simulink model "untitled"  (R2020b)
settings: Solver=ode1  StartTime=0  StopTime=max(T)  FixedStep=0.01  RelTol=1e-3
values from neighbouring files (symbols this model uses):
  H = [0 costh 0 ... (first row only)    [kalmanf_unbias.m]
  P0 = [10000 5000 5000 ... (first row only)    [Kalman.m]
  Q = [100 50 25 ... (first row only)    [Kalman.m]
  R = [10 5 5 ... (first row only)    [Kalman.m]
  x0 = zeros(3,1)    [Kalman.m]
settings Model: Creator=Stergios  LastModifiedBy=Stergios

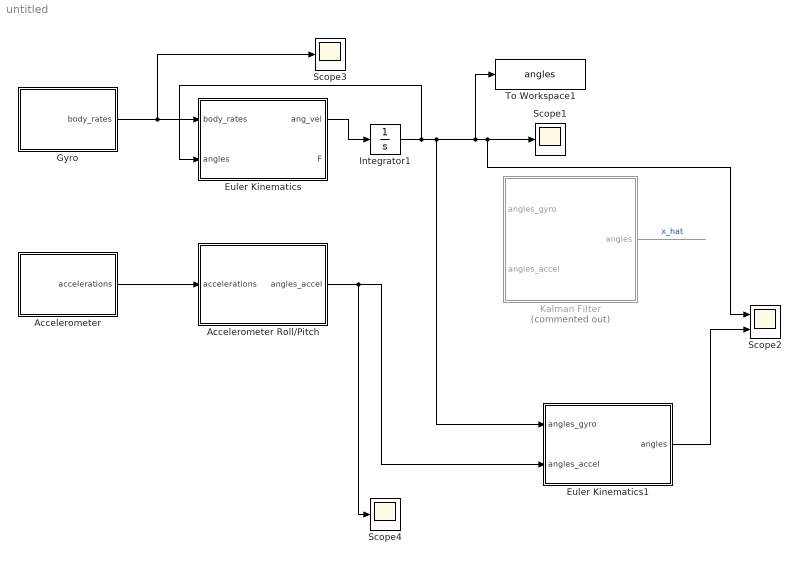
== system untitled ==
  Accelerometer : Subsystem
  Accelerometer Roll/Pitch : MATLAB Function  TreatAsAtomicUnit=on
  Euler Kinematics : MATLAB Function  TreatAsAtomicUnit=on
  Euler Kinematics1 : MATLAB Function  TreatAsAtomicUnit=on
  Gyro : Subsystem
  Integrator1 : Integrator  InitialCondition=[0 0 0]
  Kalman Filter : MATLAB Function  Commented=on  TreatAsAtomicUnit=on  mask{x0=x0, P0=P0, Q=Q, R=R, H=H}
      mask prompts: x0 "Initial State:"; P0 "Initial State Covariance Matrix:"; Q "Process Noise Covariance Matrix:"; R "Measurement Noise Covariance Matrix:"; H "Observation Matrix:"
  Scope1 : Scope
  Scope2 : Scope  NumInputPorts=2
  Scope3 : Scope
  Scope4 : Scope
  To Workspace1 : ToWorkspace  VariableName=angles  SampleTime=-1
  wires:
  Integrator1/1 -> Euler Kinematics1/1(angles_gyro), Scope1/1, Scope2/1, To Workspace1/1, Euler Kinematics/2(angles)
  Euler Kinematics/1(ang_vel) -> Integrator1/1
  Gyro/1(body_rates) -> Scope3/1, Euler Kinematics/1(body_rates)
  Accelerometer/1(accelerations) -> Accelerometer Roll/Pitch/1(accelerations)
  Kalman Filter/1(angles) -> ?  "x_hat"
  Euler Kinematics1/1(angles) -> Scope2/2
  Accelerometer Roll/Pitch/1(angles_accel) -> Scope4/1, Euler Kinematics1/2(angles_accel)

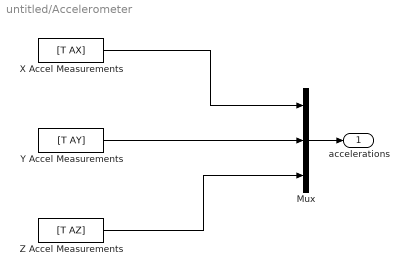
== system untitled/Accelerometer ==
  Mux : Mux  Inputs=3
  X Accel Measurements : FromWorkspace  VariableName=[T AX]
  Y Accel Measurements : FromWorkspace  VariableName=[T AY]
  Z Accel Measurements : FromWorkspace  VariableName=[T AZ]
  accelerations : Outport
  wires:
  Y Accel Measurements/1 -> Mux/2
  Z Accel Measurements/1 -> Mux/3
  Mux/1 -> accelerations/1
  X Accel Measurements/1 -> Mux/1

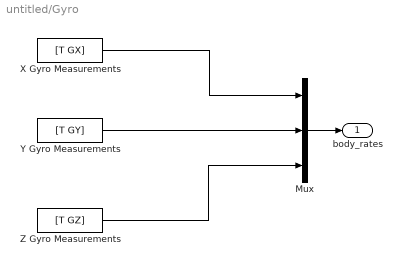
== system untitled/Gyro ==
  Mux : Mux  Inputs=3
  X Gyro Measurements : FromWorkspace  VariableName=[T GX]
  Y Gyro Measurements : FromWorkspace  VariableName=[T GY]
  Z Gyro Measurements : FromWorkspace  VariableName=[T GZ]
  body_rates : Outport
  wires:
  Mux/1 -> body_rates/1
  X Gyro Measurements/1 -> Mux/1
  Y Gyro Measurements/1 -> Mux/2
  Z Gyro Measurements/1 -> Mux/3

== matlab function untitled/Euler Kinematics ==
  data: body_rates input; ang_vel output; angles input; F output
function [ang_vel,F]=fcn(body_rates,angles)
    phi = angles(1)*pi/180;
    theta = angles(2)*pi/180;
    
    F = [1,tan(theta)*sin(phi),tan(theta)*cos(phi);
        0,cos(phi),-sin(phi);
        0,sin(phi)/cos(theta),cos(phi)/cos(theta)];

    ang_vel = F*body_rates;
end

== matlab function untitled/Accelerometer Roll//Pitch ==
  data: accelerations input; angles_accel output
function angles_accel =fcn(accelerations)
    mu = 0.01;
    angles_accel=zeros(3,1);
    angles_accel(1) = atan(accelerations(2)/(sign(accelerations(3))*sqrt(accelerations(3)^2+mu*accelerations(1)^2)))*180/pi;
    angles_accel(2) = atan(-accelerations(1)/sqrt(accelerations(2)^2+accelerations(3)^2))*180/pi;
    angles_accel(3) = 0;
    
end

== matlab function untitled/Euler Kinematics1 ==
  data: angles_gyro input; angles output; angles_accel input
function angles = fcn(angles_gyro,angles_accel)
    gain = 0.6;
    angles = gain*angles_gyro+(1-gain)*angles_accel;
end

== matlab function untitled/Kalman Filter ==
  data: angles_gyro input; angles_accel input; angles output
function angles = fcn(angles_gyro,angles_accel)
    x__ = angles_gyro;
    x_ = x__+ni;
    P_ = P0+Q;
    K = P_/(P_+R)
    x__ = x_ +K*(angles_accel-x_')';
    P__ =(eye(3)-K)*P_;
    angles = x__';

end
